simulink model "Q_3_2_Friction_Estimation"  (R2024b)
settings: Solver=VariableStepAuto  StartTime=0.0  StopTime=45  RelTol=1e-3
InitFcn:
  | load_params_inertial_case
  | PID_calculations
  | PID_Calculations_w
values from neighbouring files (symbols this model uses):
  delta_c = 1 / sqrt(2)    [PID_calculations.m]
  delta_i = 1 / sqrt(2)    [PID_calculations.m]
  K_D_w = K_P_w * T_D_w    [PID_Calculations_w.m]
  K_I_w = K_P_w / T_I_w    [PID_Calculations_w.m]
  K_P_w = DeltaK_w * cos(DeltaPhi_w)    [PID_Calculations_w.m]
  rads2rpm = 60/(2*pi)    (= 9.54929658551)    [load_params_inertial_case.m]
  rpm2rads = 2*pi/60    (= 0.10471975512)    [load_params_inertial_case.m]
  w_c = 2 * pi * 20    (= 125.663706144)    [PID_calculations.m]
undefined symbols (not defined in the file or in its folder): gbox, mot, sens, T_L_w, w_c_i
settings Model: Creator=JS  LastModifiedBy=JS

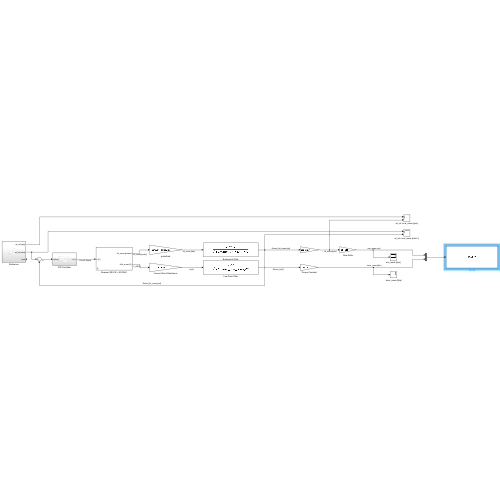
[thumbnail: Simulink's stored preview of the top-level diagram]
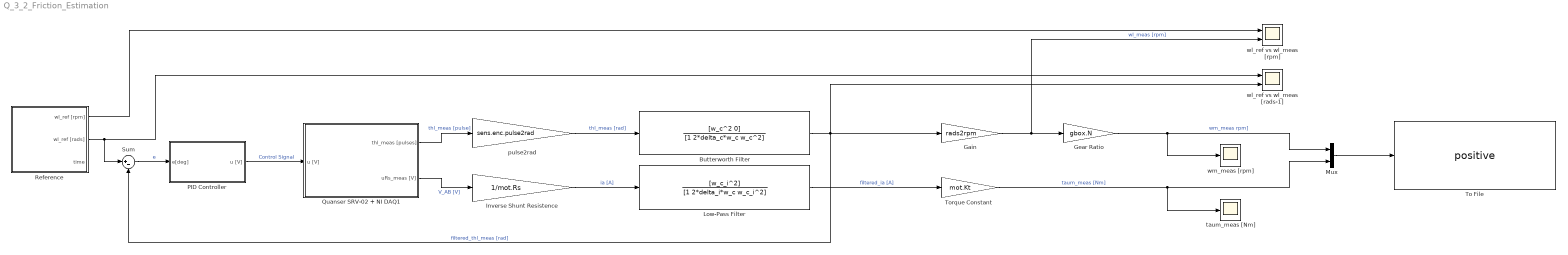
== system Q_3_2_Friction_Estimation ==
  " taum_meas [Nm]" : Scope
  Butterworth Filter : TransferFcn  Numerator=[w_c^2 0]  Denominator=[1 2*delta_c*w_c w_c^2]
  Gain : Gain  Gain=rads2rpm
  Gear Ratio : Gain  Gain=gbox.N
  Inverse Shunt Resistence : Gain  Gain=1/mot.Rs
  Low-Pass Filter : TransferFcn  Numerator=[w_c_i^2]  Denominator=[1 2*delta_i*w_c w_c_i^2]
  Mux : Mux  Inputs=2
  PID Controller : Subsystem
  Quanser SRV-02 + NI DAQ1 : Subsystem  mask(Quanser SRV-02 (with inertial load) + NI DAQ){Ts=0.001, fricType=Coulomb + viscous}
      mask prompts: Ts "NI DAQ Sample Time:"; fricType "Friction model"
      mask help: Quanser SRV-02 (with inertial load) + NI DAQ model.
      mask init:
      | %%  Sensors data
      | 
      | %   shunt resistor
      | sens.curr.Rs = 0.5;                         %   resistance [Ohm]   
      | sens.curr.uRs_std = 0.01;                   %   voltage noise standard dev [V]                           
      | sens.curr.uRs_var = sens.curr.uRs_std^2;	%   voltage noise variance [V^2]
      | 
      | %   Hewlett-Packard HEDS-5540#A06 optical encoder
      | sens.enc.ppr = 500*4;                       %   pulses per rotation
      | sens.enc.pulse2deg = 360/sens.enc.ppr;      %   [pulses] -> [deg]
      | sens.enc.pulse2rad = 2*pi/sens.enc.ppr;     %   [pulses] -> [rad]
      | sens.enc.deg2pulse = sens.enc.ppr/360;      %   [deg] -> [pulses]
      | sens.enc.rad2pulse = sens.enc.ppr/2/pi;     %   [rad] -> [pulses]
      | 
      | 
      | %%  Data acquisition board (daq) data
      | 
      | %   NI PCI-6221 DAC data
      | daq.dac.bits = 16;                                  %   resolution (bits)
      | daq.dac.fs   = 10;                                  %   full scale 
      | daq.dac.q    = 2*daq.dac.fs/(2^daq.dac.bits-1);     %	quantization
      | 
      | %   NI PCI-6221 ADC data
      | daq.adc.bits = 16;                                  %   resolution (bits)
      | daq.adc.fs   = 10;                                  %   full scale (as set in SLDRT Analog Input block)
      | daq.adc.q    = 2*daq.adc.fs/(2^daq.adc.bits-1);     %   quantization
      mask Help:
      | Riccardo Antonello (antonello@dei.unipd.it)
      | 
      | April 24, 2020
      | 
      | Dept. of Information Engineering, University of Padova
      mask TypeOptions fricType: Coulomb + viscous | Karnopp
  Reference : Subsystem
  Sum : Sum  Inputs=|+-
  To File : ToFile  Filename=positive  MatrixName=positive  SaveFormat=Timeseries
  Torque Constant : Gain  Gain=mot.Kt
  pulse2rad : Gain  Gain=sens.enc.pulse2rad
  wl_ref vs wl_meas [rads-1] : Scope  NumInputPorts=2
  wl_ref vs wl_meas [rpm] : Scope  NumInputPorts=2
  wm_meas [rpm] : Scope
  wires:
  PID Controller/1(u [V]) -> Quanser SRV-02 + NI DAQ1/1(u [V])  "Control Signal"
  Reference/1(wl_ref [rpm]) -> wl_ref vs wl_meas [rpm]/1
  Quanser SRV-02 + NI DAQ1/1(thl_meas [pulses]) -> pulse2rad/1  "thl_meas [pulse]"
  Quanser SRV-02 + NI DAQ1/2(uRs_meas [V]) -> Inverse Shunt Resistence/1  "V_AB [V]"
  Reference/2(wl_ref [rads]) -> wl_ref vs wl_meas [rads-1]/1, Sum/1
  Gear Ratio/1 -> wm_meas [rpm]/1, Mux/1  "wm_meas rpm]"
  Gain/1 -> wl_ref vs wl_meas [rpm]/2, Gear Ratio/1  "wl_meas [rpm]"
  Torque Constant/1 -> " taum_meas [Nm]"/1, Mux/2  "taum_meas [Nm]"
  pulse2rad/1 -> Butterworth Filter/1  "thl_meas [rad]"
  Butterworth Filter/1 -> Gain/1, Sum/2, wl_ref vs wl_meas [rads-1]/2  "filtered_thl_meas [rad]"
  Inverse Shunt Resistence/1 -> Low-Pass Filter/1  "ia [A]"
  Low-Pass Filter/1 -> Torque Constant/1  "filtered_ia [A]"
  Mux/1 -> To File/1
  Sum/1 -> PID Controller/1(e[deg])  "e"

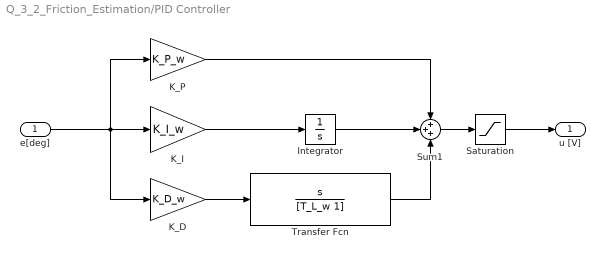
== system Q_3_2_Friction_Estimation/PID Controller ==
  e[deg] : Inport
  Integrator : Integrator  ZeroCross=off
  K_D : Gain  Gain=K_D_w
  K_I : Gain  Gain=K_I_w
  K_P : Gain  Gain=K_P_w
  Saturation : Saturate  UpperLimit=10  LowerLimit=-10
  Sum1 : Sum  Inputs=+++
  Transfer Fcn : TransferFcn  Numerator=[1 0]  Denominator=[T_L_w 1]
  u [V] : Outport
  wires:
  Sum1/1 -> Saturation/1
  e[deg]/1 -> K_D/1, K_I/1, K_P/1
  K_D/1 -> Transfer Fcn/1
  Integrator/1 -> Sum1/2
  Saturation/1 -> u [V]/1
  K_I/1 -> Integrator/1
  Transfer Fcn/1 -> Sum1/3
  K_P/1 -> Sum1/1

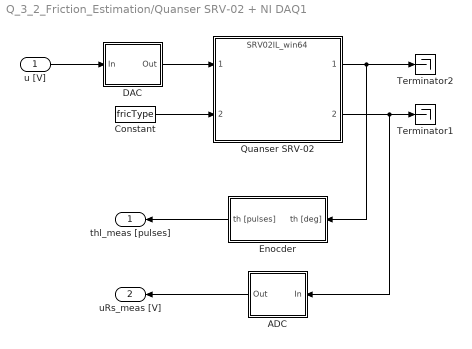
== system Q_3_2_Friction_Estimation/Quanser SRV-02 + NI DAQ1 ==
  u [V] : Inport
  ADC : Subsystem
  Constant : Constant  Value=fricType
  DAC : Subsystem
  Enocder : Subsystem
  Quanser SRV-02 : ModelReference  ModelNameDialog=SRV02IL_win64.slxp  ModelReferenceVersion=1.44  CopyOfModelProtected=on
  Terminator1 : Terminator
  Terminator2 : Terminator
  thl_meas [pulses] : Outport
  uRs_meas [V] : Outport  Port=2
  wires:
  Enocder/1(th [pulses]) -> thl_meas [pulses]/1
  ADC/1(Out) -> uRs_meas [V]/1
  DAC/1(Out) -> Quanser SRV-02/1
  Quanser SRV-02/2 -> ADC/1(In), Terminator1/1
  u [V]/1 -> DAC/1(In)
  Quanser SRV-02/1 -> Enocder/1(th [deg]), Terminator2/1
  Constant/1 -> Quanser SRV-02/2

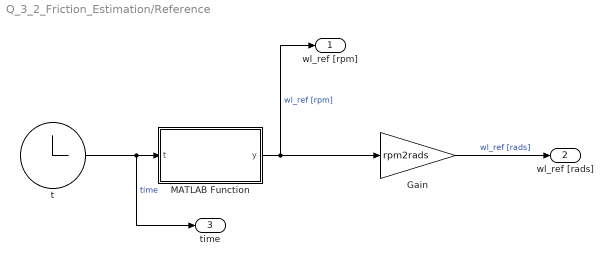
== system Q_3_2_Friction_Estimation/Reference ==
  Gain : Gain  Gain=rpm2rads
  MATLAB Function : MATLAB Function  TreatAsAtomicUnit=on
  t : Clock
  wl_ref [rpm] : Outport
  wl_ref [rads] : Outport  Port=2
  time : Outport  Port=3
  wires:
  MATLAB Function/1(y) -> wl_ref [rpm]/1, Gain/1  "wl_ref [rpm]"
  t/1 -> time/1, MATLAB Function/1(t)  "time"
  Gain/1 -> wl_ref [rads]/1  "wl_ref [rads]"

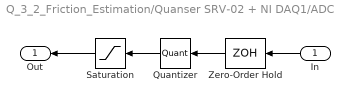
== system Q_3_2_Friction_Estimation/Quanser SRV-02 + NI DAQ1/ADC ==
  In : Inport
  Quantizer : Quantizer  QuantizationInterval=daq.adc.q
  Saturation : Saturate  UpperLimit=daq.adc.fs  LowerLimit=-daq.adc.fs
  Zero-Order Hold : ZeroOrderHold  SampleTime=Ts
  Out : Outport
  wires:
  Saturation/1 -> Out/1
  In/1 -> Zero-Order Hold/1
  Quantizer/1 -> Saturation/1
  Zero-Order Hold/1 -> Quantizer/1

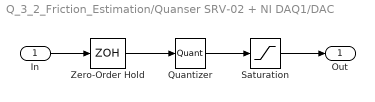
== system Q_3_2_Friction_Estimation/Quanser SRV-02 + NI DAQ1/DAC ==
  In : Inport
  Quantizer : Quantizer  QuantizationInterval=daq.dac.q
  Saturation : Saturate  UpperLimit=daq.dac.fs  LowerLimit=-daq.dac.fs
  Zero-Order Hold : ZeroOrderHold  SampleTime=Ts
  Out : Outport
  wires:
  Quantizer/1 -> Saturation/1
  In/1 -> Zero-Order Hold/1
  Zero-Order Hold/1 -> Quantizer/1
  Saturation/1 -> Out/1

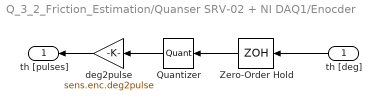
== system Q_3_2_Friction_Estimation/Quanser SRV-02 + NI DAQ1/Enocder ==
  th [deg] : Inport
  Quantizer : Quantizer  QuantizationInterval=sens.enc.pulse2deg
  Zero-Order Hold : ZeroOrderHold  SampleTime=Ts
  deg2pulse : Gain  Gain=sens.enc.deg2pulse
  th [pulses] : Outport
  wires:
  Quantizer/1 -> deg2pulse/1
  th [deg]/1 -> Zero-Order Hold/1
  Zero-Order Hold/1 -> Quantizer/1
  deg2pulse/1 -> th [pulses]/1

== matlab function Q_3_2_Friction_Estimation/Reference/MATLAB Function ==
  data: t input; y output
function y = increasing_step(t)
    step_size = 50; % Amplitude decrease per step
    step_interval = 5; % Step time interval (seconds)
    total_time = 45; % Total duration

    % Ensure first step starts at -50 at t = 0
    y = step_size * (floor(t / step_interval) + 1);

    % Hold final value at t = total_time
    if t >= total_time
        y = step_size * (floor(total_time / step_interval) + 1); % Hold final value
    end
end
